simulink model "PID_Tracking_Control"  (R2015a)
settings: Solver=ode3  StartTime=0.0  StopTime=1000  FixedStep=0.1  RelTol=1e-3
libraries: simulink x4
settings Model: Creator=Muhammad Bilal Kadri  LastModifiedBy=Muhammad Bilal Kadri
settings SolverCC: AutoInsertRateTranBlk=on

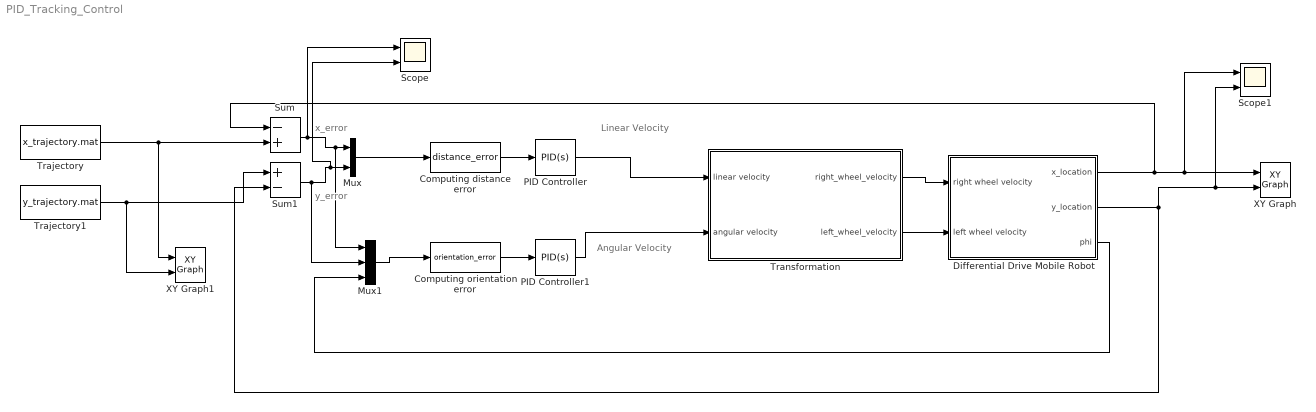
== system PID_Tracking_Control ==
  note: y_error
  note: x_error
  note: Angular Velocity
  note: Linear Velocity
  Computing distance error : MATLABFcn  MATLABFcn=distance_error  OutputDimensions=1
  Computing orientation error : MATLABFcn  MATLABFcn=orientation_error  OutputDimensions=1
  Differential Drive Mobile Robot : Subsystem  mask{R=5, L=10}
      mask prompts: R "Wheel Radius"; L "Distance between wheels"
  Mux : Mux  Inputs=2
  Mux1 : Mux  Inputs=3
  PID Controller : simulink/Continuous/PID Controller  Controller=PID  TimeDomain=Continuous-time  SampleTime=-1  IntegratorMethod=Forward Euler  FilterMethod=Forward Euler  Form=Parallel  UseFilter=on  ControllerParametersSource=internal  P=0.0504359921516874  I=0.00100836074716022  D=-0.0162580875537082  N=1.13639880092487  InitialConditionSource=internal  InitialConditionForIntegrator=0  InitialConditionForFilter=0  ExternalReset=none  LimitOutput=off  UpperSaturationLimit=inf  LowerSaturationLimit=-inf  LinearizeAsGain=on  AntiWindupMode=none  Kb=1  TrackingMode=off  Kt=1  PParamMin=[]  PParamMax=[]  IParamMin=[]  IParamMax=[]  DParamMin=[]  DParamMax=[]  NParamMin=[]  NParamMax=[]  KbParamMin=[]  KbParamMax=[]  KtParamMin=[]  KtParamMax=[]  POutMin=[]  POutMax=[]  IOutMin=[]  IOutMax=[]  DOutMin=[]  DOutMax=[]  NOutMin=[]  NOutMax=[]  KbOutMin=[]  KbOutMax=[]  KtOutMin=[]  KtOutMax=[]  IntegratorOutMin=[]  IntegratorOutMax=[]  FilterOutMin=[]  FilterOutMax=[]  SumOutMin=[]  SumOutMax=[]  SumI1OutMin=[]  SumI1OutMax=[]  SumI2OutMin=[]  SumI2OutMax=[]  SumI3OutMin=[]  SumI3OutMax=[]  SumDOutMin=[]  SumDOutMax=[]  SaturationOutMin=[]  SaturationOutMax=[]  IntegratorContinuousStateAttributes=''  IntegratorStateMustResolveToSignalObject=off  IntegratorRTWStateStorageClass=Auto  FilterContinuousStateAttributes=''  FilterStateMustResolveToSignalObject=off  FilterRTWStateStorageClass=Auto  DifferentiatorICPrevScaledInput=0  DifferentiatorOutMin=[]  DifferentiatorOutMax=[]
  PID Controller1 : simulink/Continuous/PID Controller  Controller=PID  TimeDomain=Continuous-time  SampleTime=-1  IntegratorMethod=Forward Euler  FilterMethod=Forward Euler  Form=Parallel  UseFilter=on  ControllerParametersSource=internal  P=0.000344915523931585  I=5.40874878904373e-08  D=0.479966099643471  N=3.01968832345364  InitialConditionSource=internal  InitialConditionForIntegrator=0  InitialConditionForFilter=0  ExternalReset=none  LimitOutput=off  UpperSaturationLimit=inf  LowerSaturationLimit=-inf  LinearizeAsGain=on  AntiWindupMode=none  Kb=1  TrackingMode=off  Kt=1  PParamMin=[]  PParamMax=[]  IParamMin=[]  IParamMax=[]  DParamMin=[]  DParamMax=[]  NParamMin=[]  NParamMax=[]  KbParamMin=[]  KbParamMax=[]  KtParamMin=[]  KtParamMax=[]  POutMin=[]  POutMax=[]  IOutMin=[]  IOutMax=[]  DOutMin=[]  DOutMax=[]  NOutMin=[]  NOutMax=[]  KbOutMin=[]  KbOutMax=[]  KtOutMin=[]  KtOutMax=[]  IntegratorOutMin=[]  IntegratorOutMax=[]  FilterOutMin=[]  FilterOutMax=[]  SumOutMin=[]  SumOutMax=[]  SumI1OutMin=[]  SumI1OutMax=[]  SumI2OutMin=[]  SumI2OutMax=[]  SumI3OutMin=[]  SumI3OutMax=[]  SumDOutMin=[]  SumDOutMax=[]  SaturationOutMin=[]  SaturationOutMax=[]  IntegratorContinuousStateAttributes=''  IntegratorStateMustResolveToSignalObject=off  IntegratorRTWStateStorageClass=Auto  FilterContinuousStateAttributes=''  FilterStateMustResolveToSignalObject=off  FilterRTWStateStorageClass=Auto  DifferentiatorICPrevScaledInput=0  DifferentiatorOutMin=[]  DifferentiatorOutMax=[]
  Scope : Scope  NumInputPorts=2
      settings: YMin=-5~-5  YMax=5~5
  Scope1 : Scope  NumInputPorts=2
      settings: YMin=0~-6500  YMax=90000~5000
  Sum : Sum  Inputs=-+  InputSameDT=on
  Sum1 : Sum  Inputs=+-
  Trajectory : FromFile  FileName=x_trajectory.mat  SampleTime=1
  Trajectory1 : FromFile  FileName=y_trajectory.mat  SampleTime=1
  Transformation : Subsystem  mask{R=5, L=10}
      mask prompts: R "Wheel Radius"; L "Distance between wheels"
  XY Graph : simulink/Sinks/XY Graph  xmin=0  xmax=30  ymin=0  ymax=30  st=1
  XY Graph1 : simulink/Sinks/XY Graph  xmin=0  xmax=30  ymin=0  ymax=30  st=1
  wires:
  PID Controller/1 -> Transformation/1(linear velocity)
  PID Controller1/1 -> Transformation/2(angular velocity)
  Transformation/1(right_wheel_velocity) -> Differential Drive Mobile Robot/1(right wheel velocity)
  Transformation/2(left_wheel_velocity) -> Differential Drive Mobile Robot/2(left wheel velocity)
  Computing distance error/1 -> PID Controller/1
  Computing orientation error/1 -> PID Controller1/1
  Differential Drive Mobile Robot/1(x_location) -> Sum/1, Scope1/1, XY Graph/1
  Trajectory/1 -> XY Graph1/1, Sum/2
  Sum/1 -> Scope/1, Mux1/1, Mux/1
  Trajectory1/1 -> XY Graph1/2, Sum1/1
  Sum1/1 -> Mux1/2, Scope/2, Mux/2
  Mux/1 -> Computing distance error/1
  Mux1/1 -> Computing orientation error/1
  Differential Drive Mobile Robot/3(phi) -> Mux1/3
  Differential Drive Mobile Robot/2(y_location) -> Sum1/2, Scope1/2, XY Graph/2

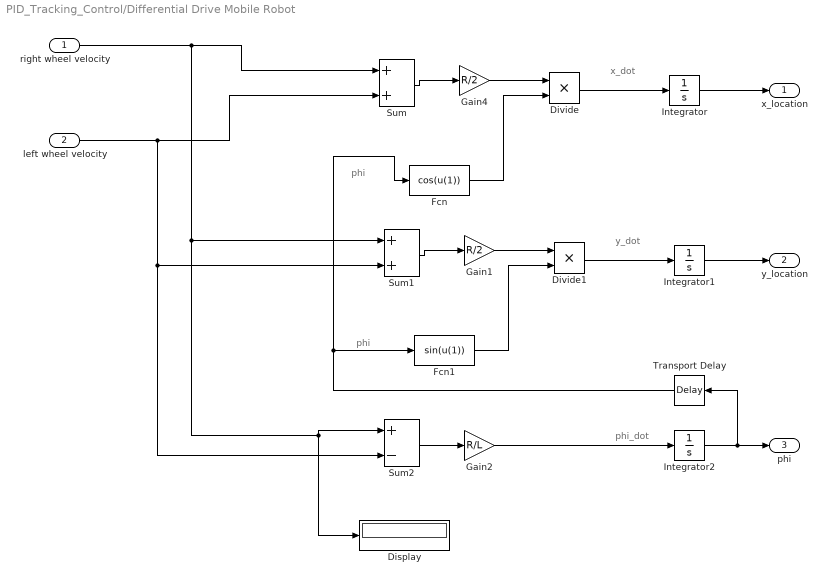
== system PID_Tracking_Control/Differential Drive Mobile Robot ==
  note: phi
  note: x_dot
  note: phi
  note: y_dot
  note: phi_dot
  right wheel velocity : Inport
  left wheel velocity : Inport  Port=2
  Display : Display
  Divide : Product  Inputs=**
  Divide1 : Product  Inputs=**
  Fcn : Fcn  Expr=cos(u(1))
  Fcn1 : Fcn  Expr=sin(u(1))
  Gain1 : Gain  Gain=R/2
  Gain2 : Gain  Gain=R/L
  Gain4 : Gain  Gain=R/2
  Integrator : Integrator
  Integrator1 : Integrator
  Integrator2 : Integrator
  Sum : Sum
  Sum1 : Sum
  Sum2 : Sum  Inputs=+-
  Transport Delay : TransportDelay
  x_location : Outport
  y_location : Outport  Port=2
  phi : Outport  Port=3
  wires:
  Sum/1 -> Gain4/1
  Divide/1 -> Integrator/1
  Integrator/1 -> x_location/1
  Gain4/1 -> Divide/1
  Fcn/1 -> Divide/2
  Transport Delay/1 -> Fcn/1, Fcn1/1
  Sum1/1 -> Gain1/1
  Divide1/1 -> Integrator1/1
  Integrator1/1 -> y_location/1
  Gain1/1 -> Divide1/1
  Fcn1/1 -> Divide1/2
  right wheel velocity/1 -> Display/1, Sum2/1, Sum1/1, Sum/1
  left wheel velocity/1 -> Sum2/2, Sum1/2, Sum/2
  Sum2/1 -> Gain2/1
  Gain2/1 -> Integrator2/1
  Integrator2/1 -> Transport Delay/1, phi/1

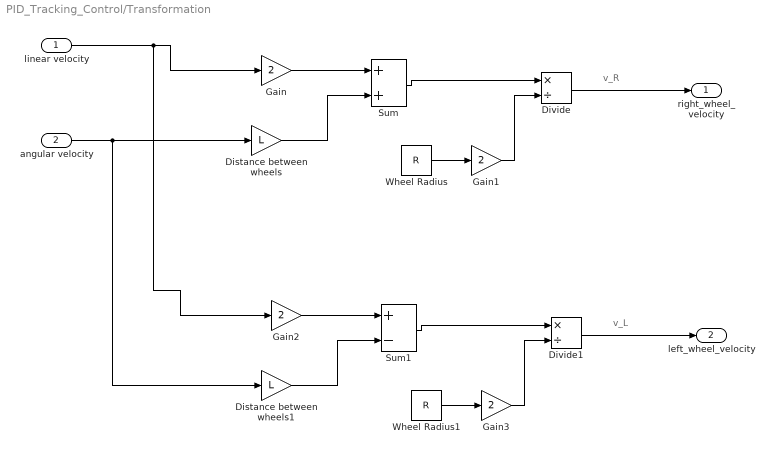
== system PID_Tracking_Control/Transformation ==
  note: v_R
  note: v_L
  linear velocity : Inport
  angular velocity : Inport  Port=2
  Distance between wheels : Gain  Gain=L
  Distance between wheels1 : Gain  Gain=L
  Divide : Product  Inputs=*/
  Divide1 : Product  Inputs=*/
  Gain{,1..3} (4 alike) : Gain  Gain=2
  Sum : Sum
  Sum1 : Sum  Inputs=+-
  Wheel Radius : Constant  Value=R
  Wheel Radius1 : Constant  Value=R
  right_wheel_velocity : Outport
  left_wheel_velocity : Outport  Port=2
  wires:
  Sum/1 -> Divide/1
  Gain1/1 -> Divide/2
  Distance between wheels/1 -> Sum/2
  Gain/1 -> Sum/1
  Wheel Radius/1 -> Gain1/1
  Divide/1 -> right_wheel_velocity/1
  Sum1/1 -> Divide1/1
  Gain3/1 -> Divide1/2
  Distance between wheels1/1 -> Sum1/2
  Gain2/1 -> Sum1/1
  Wheel Radius1/1 -> Gain3/1
  Divide1/1 -> left_wheel_velocity/1
  angular velocity/1 -> Distance between wheels1/1, Distance between wheels/1
  linear velocity/1 -> Gain2/1, Gain/1
